simulink model "Simulacao"  (Simulink 8.2)
settings: Solver=ode4  SolverMode=SingleTasking  StartTime=0.0  StopTime=1000  FixedStep=0.01  RelTol=1e-3
InitFcn:
  | Main_Simulink;
values from neighbouring files (symbols this model uses):
  C = [1 0]    [MatrizesDeEstado.m]
  Cstate = eye(n)    [MatrizesDeEstado.m]
  Dstate = 0*Cstate(:,n)    [MatrizesDeEstado.m]
  T = 1    [Main.m]
undefined symbols (not defined in the file or in its folder): A, B, xk0
undefined symbols (not defined in the file): H, R, rho, S, Umax
settings Model: Creator=Kawakami  LastModifiedBy=Eduardo
settings DataIOCC: LimitDataPoints=off  SaveOutput=off  SaveTime=off  TimeSaveName=t  SignalLoggingName=sigsOut
settings OptimizationCC: BooleanDataType=off
settings DebuggingCC: SaveWithParameterizedLinksMsg=none  SignalResolutionControl=TryResolveAllWithWarning  SolverPrmCheckMsg=none  MultiTaskDSMMsg=warning  MultiTaskCondExecSysMsg=none
settings HardwareCC: TargetUnknown=on
settings RTWCC: IncludeERTFirstTime=on

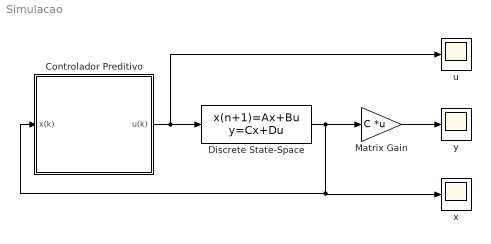
== system Simulacao ==
  "Controlador Preditivo  " : Subsystem  mask{A=A, B=B, H=H, S=S, R=R, Umax=Umax, T=T, rho=rho}
      mask prompts: A "Matriz Agregada A"; B "Matriz Agregada B"; H "H (imagem da Aeq)"; S "S (custo quadrático)"; R "R (custo quadrático)"; Umax "Input Max"; T "T (passo da simulação)"; rho "rho (peso para o Gamma)"
  Discrete State-Space : DiscreteStateSpace  A=A{1}  B=B{1}  C=Cstate  D=Dstate  X0=xk0  SampleTime=T
  Matrix Gain : Gain  Gain=C  Multiplication=Matrix(K*u)  SampleTime=T  SaturateOnIntegerOverflow=on  OutDataTypeStr=Inherit: Same as input  ParamDataTypeStr=Inherit: Same as input
  u : Scope
      settings: TimeRange=10  YMin=0.065  YMax=0.1075
  x : Scope
      settings: TimeRange=100  YMin=-191.5000000000001  YMax=48.49999999999989
  y : Scope
      settings: TimeRange=100  YMin=-191.5000000000001  YMax=48.49999999999989  SaveName=ScopeData2
  wires:
  "Controlador Preditivo  "/1(u(k)) -> Discrete State-Space/1, u/1
  Discrete State-Space/1 -> Matrix Gain/1, x/1, "Controlador Preditivo  "/1(x(k))
  Matrix Gain/1 -> y/1

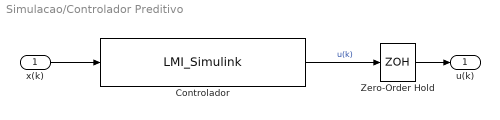
== system Simulacao/Controlador Preditivo   ==
  x(k) : Inport
  Controlador : S-Function  FunctionName=LMI_Simulink  Parameters=A, B, S, R, Smeio, Rmeio, H, Umax, rho, T  EnableBusSupport=off
  Zero-Order Hold : ZeroOrderHold  SampleTime=T
  u(k) : Outport
  wires:
  Zero-Order Hold/1 -> u(k)/1
  Controlador/1 -> Zero-Order Hold/1  "u(k)"
  x(k)/1 -> Controlador/1
